simulink model "test_com_SensorFusion_SF_D4_ukf"  (R2019b)
settings: Solver=FixedStepDiscrete  StartTime=0  StopTime=stop  FixedStep=0.001  RelTol=1e-3
undefined symbols (not defined in the file or in its folder): breakpoints_camber_posZ, breakpoints_camber_RollAngle, BxTM, ByTM, camber_posZ_rear, camber_RollAngle_front, camber_RollAngle_rear, CxTM, CyTM, enable_kalman_standing, enable_simpleTireLoad_pGL, enable_v2o_direct, g, gamma_stat_front, gamma_stat_rear, gearbox_ratio, l_F, l_R, m_sprung, m_unsprung_quarter, mag_calib_front_center, mag_calib_front_compmatrix, mag_calib_rear_center, mag_calib_rear_compmatrix, should_be_in_theSensorFusion, switch_lat_accel_tireloadestimE8, switch_rocker_direction_FL, switch_rocker_direction_FR, switch_rocker_direction_RL, switch_rocker_direction_RR, switch_VelYcalculation_pSF, testStart_VelX_pSF, testVelY_pSF, tire_r_dyn, track_angle_front, track_width_front, track_width_rear, v2o_x, wheel_kinematics_breakpoints, wheel_kinematics_FL_data, wheel_kinematics_FR_data, wheelbase, x9DFrontX, x9DFrontY, x9DRearX, x9DRearY
libraries: SignalProcessingSensorFusionLib x30, simulink x9
(part 9 of 9)

== matlab function test_com_SensorFusion_SF_D4_ukf/Subsystem14/SensorFusion_D4/SiDes Testgelände ==
  data: measurements_nb input; easyYawRate_out output; x input; easyYawAngle_out output; easyPos_out output; wheelbase parameter; delta input; dt input; YawRateBySteer output
function [easyYawRate_out,easyYawAngle_out,easyPos_out,YawRateBySteer] = fcn(measurements_nb,x,wheelbase, delta,dt)

persistent easyPosX easyPosY easyYawAngle easyYawRate
persistent temp


if isempty(temp)
    temp=420;
       

    easyPosX =single(0);
    easyPosY =single(0);
    easyYawAngle =single(0);
    easyYawRate  =single(0);
end



PosX=x(1);
VelX=x(2);
AccX=x(3);
PosY=x(4);
VelY=x(5);
AccY=x(6);
PosZ=x(7);
VelZ=x(8);
AccZ=x(9);
RollAngle=x(10);
RollRate=x(11);
RollAcc=x(12);
PitchAngle=x(13);
PitchRate=x(14);
PitchAcc=x(15);
YawAngle=x(16);
YawRate=x(17);
YawAcc=x(18);
WheelSpeed_FL=x(19);
WheelSpeed_FR=x(20);
WheelSpeed_RL=x(21);
WheelSpeed_RR=x(22);

    WheelSpeeds_nb=     single(zeros(4,1));
    RockerAngle_nb=     single(zeros(4,1));

v2o_VelX_nb=            measurements_nb(1);
v2o_VelY_nb=            measurements_nb(2);
v2o_SlipAngle_nb=       measurements_nb(3);
x9D_Front_AccX_nb=      measurements_nb(4);
x9D_Front_AccY_nb=      measurements_nb(5);
x9D_Front_AccZ_nb=      measurements_nb(6);     %Gravitation berücksichtigen ???
x9D_Front_RollRate_nb=  measurements_nb(7);
x9D_Front_PitchRate_nb= measurements_nb(8);
x9D_Front_YawRate_nb=   measurements_nb(9);
x9D_Rear_AccX_nb=       measurements_nb(10);
x9D_Rear_AccY_nb=       measurements_nb(11);
x9D_Rear_AccZ_nb=       measurements_nb(12);    %Gravitation berücksichtigen ???
x9D_Rear_RollRate_nb=   measurements_nb(13);
x9D_Rear_PitchRate_nb=  measurements_nb(14);
x9D_Rear_YawRate_nb=    measurements_nb(15);
WheelSpeeds_nb(1)=      measurements_nb(16);
WheelSpeeds_nb(2)=      measurements_nb(17);
WheelSpeeds_nb(3)=      measurements_nb(18);
WheelSpeeds_nb(4)=      measurements_nb(19);
RockerAngle_nb(1)=      measurements_nb(20);
RockerAngle_nb(2)=      measurements_nb(21);
RockerAngle_nb(3)=      measurements_nb(22);
RockerAngle_nb(4)=      measurements_nb(23);

YawRate_factor=1.167;

easyYawRate=    (1/3)*(x9D_Front_YawRate_nb+x9D_Rear_YawRate_nb);
YawRateBySteer=(delta*VelX/wheelbase);
easyYawAngle=easyYawAngle+dt*easyYawRate;
easyPosX=easyPosX+cos(easyYawAngle*YawRate_factor)*dt*VelX-sin(easyYawAngle*YawRate_factor)*dt*VelY;
easyPosY=easyPosY+sin(easyYawAngle*YawRate_factor)*dt*VelX+cos(easyYawAngle*YawRate_factor)*dt*VelY;


easyYawRate_out=easyYawRate;
easyYawAngle_out=easyYawAngle;
easyPos_out=[easyPosX;easyPosY];

== matlab function test_com_SensorFusion_SF_D4_ukf/Subsystem14/SensorFusion_D4/Sturzberechnung/MATLAB Function ==
  data: PosZ input; Camber_PosZ_front output; Camber_PosZ_rear output
function [Camber_PosZ_front, Camber_PosZ_rear] = fcn(PosZ)
Camber_PosZ_front=max(interp1([-25 -22.50 -20.00 -17.50 -15.00 -12.50 -10.00 -7.50 ...
    -5.00 -2.50 0.00 2.50 5.00 7.50 10.00 12.50 15.00 17.50 20.00 22.50 25.00 ], ...
    [-0.83 -0.74 -0.65 -0.56 -0.47 -0.39 -0.30 -0.23 -0.15 -0.07 0.00 0.07 0.14 0.20 ...
    0.27 0.33 0.39 0.44 0.50 0.55 0.60], PosZ,'spline'));
Camber_PosZ_rear=max(interp1([-25 -22.50 -20.00 -17.50 -15.00 -12.50 -10.00 -7.50 ...
    -5.00 -2.50 0.00 2.50 5.00 7.50 10.00 12.50 15.00 17.50 20.00 22.50 25.00],...
    [-0.64 -0.57 -0.50 -0.44 -0.37 -0.30 -0.24 -0.18 -0.12 -0.06 0.00 0.06 0.11 ...
    0.17 0.22 0.27 0.32 0.37 0.41 0.46 0.50], PosZ,'spline'));

end

== matlab function test_com_SensorFusion_SF_D4_ukf/Subsystem14/SensorFusion_D4/Sturzberechnung/MATLAB Function1 ==
  data: Camber_RollAngle_front output; Camber_RollAngle_rear output; RollAngle input
function [Camber_RollAngle_front, Camber_RollAngle_rear]= fcn (RollAngle)
Camber_RollAngle_front=max(interp1([-1.50 -1.35 -1.20 -1.05 -0.90 -0.75 -0.60 -0.45 -0.30 -0.15 0.00 ...
0.15 0.30 0.45 0.60 0.75 0.90 1.05 1.20 1.35 1.50], ...
    [1.02 0.92 0.82 0.72 0.62 0.52 0.42 0.31 0.21 0.11 0.00 -0.11 -0.21 -0.32 -0.43 -0.53 -0.64 ...
-0.75 -0.86 -0.97 -1.08], RollAngle,'spline'));
Camber_RollAngle_rear=max(interp1([-1.50 -1.35 -1.20 -1.05 -0.90 -0.75 -0.60 -0.45 -0.30 -0.15 0.00 ...
0.15 0.30 0.45 0.60 0.75 0.90 1.05 1.20 1.35 1.50],...
    [1.11 1.00 0.89 0.78 0.67 0.56 0.45 0.34 0.23 0.11 0.00 -0.12 -0.23 -0.35 -0.46 -0.58 ...
-0.70 -0.81 -0.93 -1.05 -1.17], RollAngle,'spline'));
end

== matlab function test_com_SensorFusion_SF_D4_ukf/Subsystem14/SensorFusion_D4/TireModel_simplePacejka1 ==
  data: TireLoad input size=4; TireSlipLong input size=4; TireLoadEff output; TireForceLong output size=4; TireSlipAngle input size=4; mux_nominal input; TireForceLat output size=4; l_F parameter; l_R parameter; wheelbase parameter; m_unsprung_quarter parameter; m_sprung parameter; BxTM parameter; ByTM parameter; CyTM parameter; CxTM parameter; g parameter
function [TireLoadEff, TireForceLong, TireForceLat] = TireModel_simplePacejka(TireLoad, TireSlipLong, TireSlipAngle, ...
    mux_nominal, l_F, l_R, wheelbase, m_unsprung_quarter, m_sprung, BxTM, ByTM, CyTM, CxTM, g)
%% set variables
Fz = TireLoad;
s_long = TireSlipLong;
s_lat = tan(TireSlipAngle); % sin???
dim_wheel = size(TireLoad);

Fx_eff = zeros(dim_wheel);
Fy_eff = zeros(dim_wheel);
Fxy_res  = zeros(dim_wheel);

e = 0.001;

%% set parameters

ez = 0.05; %0.05 richtwert dictonary
mu_x = mux_nominal;   % aus settings herführen
mu_y = 1.6;   % oder eins? 


%% calculate 
s_res = sqrt(s_long.^2 + s_lat.^2); % nominated total tire slips

Fznull_FL= 0.5*g*l_R/wheelbase*m_sprung+g*m_unsprung_quarter;
Fznull_FR= 0.5*g*l_R/wheelbase*m_sprung+g*m_unsprung_quarter;
Fznull_RL= 0.5*g*l_F/wheelbase*m_sprung+g*m_unsprung_quarter;
Fznull_RR= 0.5*g*l_F/wheelbase*m_sprung+g*m_unsprung_quarter;
Fz0=[Fznull_FL; Fznull_FR; Fznull_RL; Fznull_RR];

Fz_eff = Fz.*(1-ez*(Fz./Fz0).^2); % effective tire loads for mu
Dx = Fz_eff*mu_x; % D-terms for long. in Pacejka
Dy = Fz_eff*mu_y; % D-terms for lat. in Pacejka

Fx_stat = Fz_eff*mu_x.* sin( CxTM* atan(BxTM*s_res./mu_x) ); % pure long. tire forces
Fy_stat = Fz_eff*mu_y.* sin( CyTM* atan(ByTM*s_res./mu_y) ); % pure lat. tire forces
% Fx_stat = D_*sin( C_ * atan(B_*s_ - E_*(B_*s_-atan(B_*s_))) ) - sv;
% Fx_stat = D_*sin( C_ * atan(B_*s_ - E_*(B_*s_-atan(B_*s_))) ) - sv;

% combine long. lat. forces
for i = 1:numel(TireLoad)
    if s_res(i) == 0
        Fx_eff(i) = 0;
        Fy_eff(i) = 0;
    else
        Fxy_res(i) = sqrt( (s_long(i)^2*Fx_stat(i)^2+s_lat(i)^2*Fy_stat(i)^2)/(s_res(i)^2) );
        Fx_eff(i) = Fxy_res(i) *(s_long(i)/s_res(i)); % effective long. tire forces
        Fy_eff(i) = Fxy_res(i) *(s_lat(i)/s_res(i)); % effective lat. tire forces
    end
end

% Fxy_res = Fz_eff*mu;

TireLoadEff = double(Fz_eff);
TireForceLong = double(Fx_stat); %Fx_eff;
TireForceLat = double(Fy_stat);%Fy_eff;
end

== matlab function test_com_SensorFusion_SF_D4_ukf/Subsystem14/SensorFusion_D4/simpleTireLoadEstimation/MATLAB Function ==
  data: a_x input; F_z_vl output; a_y input; F_z_vr output; F_z_hl output; F_z_hr output
function [F_z_vl, F_z_vr, F_z_hl, F_z_hr] = Radlast_Beschleunigung_e9_SAE(a_x, a_y)
m=240;
g=9.81;
l=1.540;
l_v=0.796;
l_h=l-l_v;
h_s=0.2648;
b_v=0.6*2;
b_h=0.6*2;
F_z_vl=single(0);
F_z_vr=single(0);
F_z_hl=single(0);
F_z_hr=single(0);
 %m=Fahrzeugmasse; h_s= Schwerpunktshöhe (von SP zu Anbindung von Rods an Radträger); l_h= Abstand von HA zu
 %SP; l_v=Radstand von VA zum SP l=Radstand; a_x=Beschleunigung in x-Richtung; a_y=Beschleunigung
 %in y-Richtung; b_v=Spurbreite vorne;b_h=Spurbreite hinten; 
 
 %EDITIERT, so dass Vorzeichen vor h_s*a_y/(b_v*g) jeweils getauscht wurde

m_ges_f= m * (l-l_v)/l;
m_ges_r= m * l_v/l;
Delta_TireLoad_x = m * (h_s/(2*l))*a_x; %die 2 hier ist in E7 Radlastschätzer nicht so drin
%{ TireLoad = [...
%    m_ges_f *(0.5*g + (h_s/b_v)* a_y) - Delta_TireLoad_x ...
%    m_ges_f *(0.5*g - (h_s/b_v)* a_y) - Delta_TireLoad_x ...
%    m_ges_r *(0.5*g + (h_s/b_h)* a_y) + Delta_TireLoad_x ...
%    m_ges_r *(0.5*g - (h_s/b_h)* a_y) + Delta_TireLoad_x];
%}

SiL_WheelStates = [ ...
    m*(l_h*g-h_s*a_x)*(0.5+(h_s*a_y/(b_v*g)))/l;
    m*(l_h*g-h_s*a_x)*(0.5-(h_s*a_y/(b_v*g)))/l;
    m*(l_v*g+h_s*a_x)*(0.5+(h_s*a_y/(b_h*g)))/l;
    m*(l_v*g+h_s*a_x)*(0.5-(h_s*a_y/(b_h*g)))/l
    ];
if SiL_WheelStates(1)<0
    F_z_vl = single(0);
else
    F_z_vl = SiL_WheelStates(1);
end

if SiL_WheelStates(2)<0
    F_z_vr = single(0);
else
    F_z_vr = SiL_WheelStates(2);
end

if SiL_WheelStates(3)<0
    F_z_hl = single(0);
else
    F_z_hl = SiL_WheelStates(3);
end

if SiL_WheelStates(4)<0
    F_z_hr = single(0);
else
    F_z_hr = SiL_WheelStates(4);
end

end

== matlab function test_com_SensorFusion_SF_D4_ukf/Subsystem14/SensorFusion_D4/simpleTireLoadEstimation/MATLAB Function4 ==
  data: AccX input; AccX_out output
function AccX_out   = kalman(AccX)
persistent x P

if isempty(P)
    P=single(0);
    x=single(0);
end
Q=0.00001;
A=1;


P = A*P*A' + Q;                 % covariance matrix update
				  


K_tmp = P/(P+1);

x = x + K_tmp*(AccX-x);
P = (1 - K_tmp)*P;

AccX_out=x;
end
